simulink model "E5_G1_real"  (R2021b)
settings: Solver=VariableStepAuto  StartTime=0.0  StopTime=1  RelTol=1e-3
settings Model: Creator=new  LastModifiedBy=new

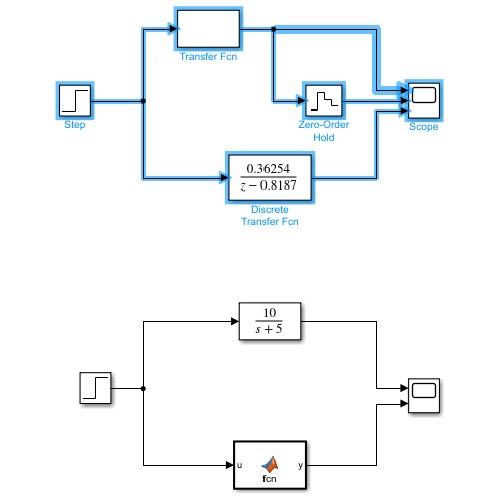
[thumbnail: Simulink's stored preview of the top-level diagram]
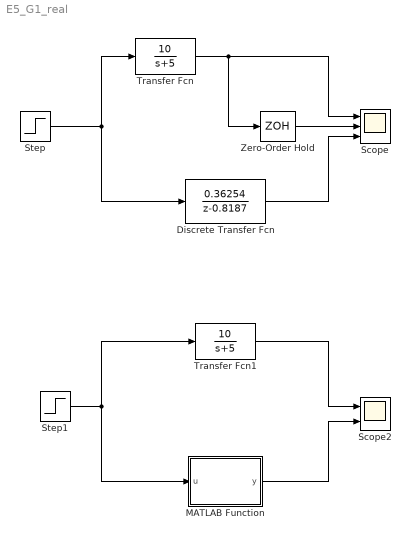
== system E5_G1_real ==
  Discrete Transfer Fcn : DiscreteTransferFcn  Numerator=[0.36254]  Denominator=[1 -0.8187]  SampleTime=0.04
  MATLAB Function : MATLAB Function  TreatAsAtomicUnit=on  SystemSampleTime=0.04
  Scope : Scope  NumInputPorts=3
  Scope2 : Scope  NumInputPorts=2
  Step : Step  Time=0  SampleTime=0
  Step1 : Step  Time=0  SampleTime=0
  Transfer Fcn : TransferFcn  Numerator=[10]  Denominator=[1 5]
  Transfer Fcn1 : TransferFcn  Numerator=[10]  Denominator=[1 5]
  Zero-Order Hold : ZeroOrderHold  SampleTime=0.04
  wires:
  Step/1 -> Discrete Transfer Fcn/1, Transfer Fcn/1
  Zero-Order Hold/1 -> Scope/2
  Discrete Transfer Fcn/1 -> Scope/3
  Transfer Fcn/1 -> Scope/1, Zero-Order Hold/1
  Transfer Fcn1/1 -> Scope2/1
  Step1/1 -> MATLAB Function/1(u), Transfer Fcn1/1
  MATLAB Function/1(y) -> Scope2/2

== matlab function E5_G1_real/MATLAB Function ==
  data: u input; y output
function y = fcn(u)
    persistent u0 u1 y0 y1
    
    if isempty(u0)
        u1=0;u0=0;y1=0;y0=0;
    end
    
    u1=u0;y1=y0;
    u0=u;
    y=0.36254*u1+0.8187*y1;
    y0=y;
